simulink model "Spring_mass_damper_system (2)"  (R2019a)
settings: Solver=VariableStepAuto  StartTime=0.0  StopTime=10  MaxStep=0.01  RelTol=1e-3
model workspace (MAT data in the model file):
  M = 10
  b = 50
  k = 100
settings Model: Creator=91839  LastModifiedBy=Shubhada
settings DataIOCC: ExternalInput=data  LoadExternalInput=on  SaveFormat=Array  DSMLogging=off  ReturnWorkspaceOutputs=off
settings DebuggingCC: SFMachineParentedDataDiag=error

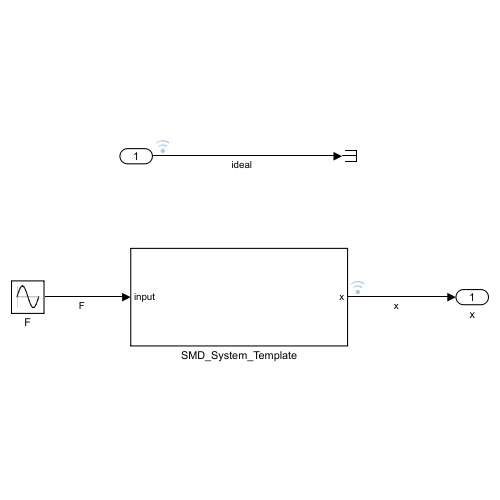
[thumbnail: Simulink's stored preview of the top-level diagram]
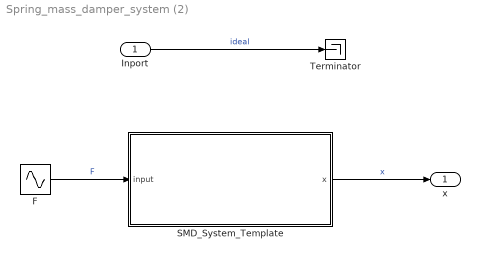
== system Spring_mass_damper_system (2) ==
  Inport : Inport
  F : Sin  SampleTime=0
  SMD_System_Template : Subsystem
  Terminator : Terminator
  x : Outport
  wires:
  Inport/1 -> Terminator/1  "ideal"
  F/1 -> SMD_System_Template/1(input)  "F"
  SMD_System_Template/1(x) -> x/1  "x"

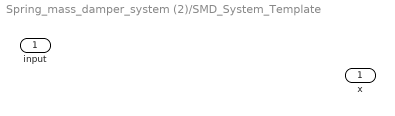
== system Spring_mass_damper_system (2)/SMD_System_Template ==
  input : Inport
  x : Outport
